simulink model "triad_estimator_test"  (R2018b)
settings: Solver=VariableStepAuto  StartTime=0.0  StopTime=10.0  RelTol=1e-3
libraries: sharedtransform x2, Triad_lib x1
settings Model: Creator=Taylor  LastModifiedBy=Taylor

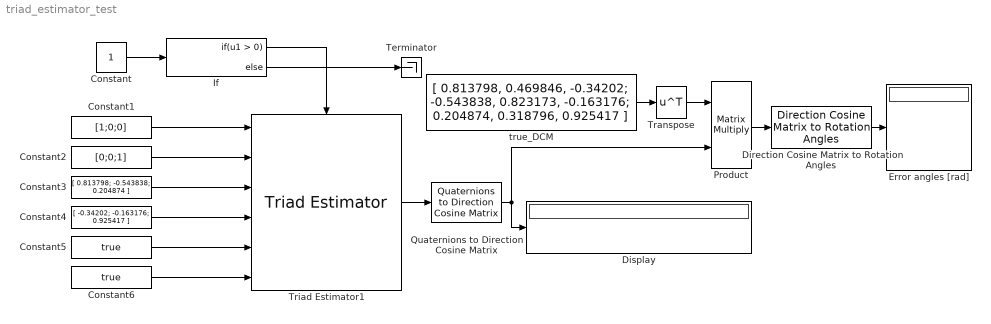
== system triad_estimator_test ==
  Constant : Constant
  Constant1 : Constant  Value=[1;0;0]
  Constant2 : Constant  Value=[0;0;1]
  Constant3 : Constant  Value=[ 0.813798; -0.543838; 0.204874 ]
  Constant4 : Constant  Value=[ -0.34202; -0.163176; 0.925417 ]
  Constant5 : Constant  Value=true
  Constant6 : Constant  Value=true
  Direction Cosine Matrix to Rotation Angles : sharedtransform/Direction Cosine Matrix to Rotation Angles  rotationOrder=ZYX  aMode=aMode  action=None  tolerance=eps(2)
      settings: SourceProductName=Aerospace Blockset  SourceProductBaseCode=AE
  Display : Display
  Error angles [rad] : Display
  If : If
  Product : Product  Multiplication=Matrix(*)
  Quaternions to Direction Cosine Matrix : sharedtransform/Quaternions to  Direction Cosine Matrix  aMode=aMode
      settings: SourceProductName=Aerospace Blockset  SourceProductBaseCode=AE
  Terminator : Terminator
  Transpose : Math  Operator=transpose  SaturateOnIntegerOverflow=on
  Triad Estimator1 : Triad_lib/Triad Estimator  SystemSampleTime=-1
  true_DCM : Constant  Value=[ 0.813798, 0.469846, -0.34202; -0.543838, 0.823173, -0.163176; 0.204874, 0.318796, 0.925417 ]
  wires:
  Constant1/1 -> Triad Estimator1/1
  Constant2/1 -> Triad Estimator1/2
  Constant3/1 -> Triad Estimator1/3
  Constant4/1 -> Triad Estimator1/4
  Constant6/1 -> Triad Estimator1/6
  Constant5/1 -> Triad Estimator1/5
  Triad Estimator1/1 -> Quaternions to Direction Cosine Matrix/1
  Constant/1 -> If/1
  If/1 -> Triad Estimator1/Action
  If/2 -> Terminator/1
  true_DCM/1 -> Transpose/1
  Quaternions to Direction Cosine Matrix/1 -> Product/2, Display/1
  Transpose/1 -> Product/1
  Product/1 -> Direction Cosine Matrix to Rotation Angles/1
  Direction Cosine Matrix to Rotation Angles/1 -> Error angles [rad]/1
